simulink model "Traffic_Light_Final"  (R2016a)
settings: Solver=FixedStepDiscrete  StartTime=0.0  StopTime=inf  RelTol=1e-3
model workspace (MAT data in the model file):
  cs : Simulink.ConfigSet (value not decoded)
settings Model: Creator=LEGION  LastModifiedBy=LEGION
settings RTWCC: GenCodeOnly=on

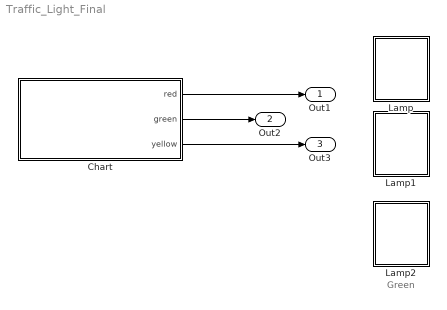
== system Traffic_Light_Final ==
  note: Green
  Chart : Stateflow chart  TreatAsAtomicUnit=on
  Lamp : Subsystem  DialogController=hmiCreateDDGDialog  IsWebBlock=on  mask(MWDashboardBlock){webBlockId=428b715c-2ac2-4c13-9f82-52b56b46ff5f, webBlockType=lamp, ShowInLibBrowser=on, ShowInitialText=on, HMISrcModelName=Traffic_Light_Final}
      mask prompts: webBlockType "WebBlock Type"; HMISrcModelName "Source Model"
      mask Help: helpview([docroot '/mapfiles/simulink.map'], 'hmi_lamp')
      mask Display:
      | if strcmp(get_param(bdroot(gcb),'BlockDiagramType'), 'library')
      |     image([(matlabroot) '/toolbox/simulink/hmi/icons/Lamp.png']);
      | end
  Lamp1 : Subsystem  DialogController=hmiCreateDDGDialog  IsWebBlock=on  mask(MWDashboardBlock){webBlockId=336aa306-1682-41f2-8291-8de665dc678f, webBlockType=lamp, ShowInLibBrowser=on, ShowInitialText=on, HMISrcModelName=Traffic_Light_Final}
      mask prompts: webBlockType "WebBlock Type"; HMISrcModelName "Source Model"
      mask Help: helpview([docroot '/mapfiles/simulink.map'], 'hmi_lamp')
      mask Display:
      | if strcmp(get_param(bdroot(gcb),'BlockDiagramType'), 'library')
      |     image([(matlabroot) '/toolbox/simulink/hmi/icons/Lamp.png']);
      | end
  Lamp2 : Subsystem  DialogController=hmiCreateDDGDialog  IsWebBlock=on  mask(MWDashboardBlock){webBlockId=cc7363f7-3161-4256-ad36-8951f7864fbc, webBlockType=lamp, ShowInLibBrowser=on, ShowInitialText=on, HMISrcModelName=Traffic_Light_Final}
      mask prompts: webBlockType "WebBlock Type"; HMISrcModelName "Source Model"
      mask Help: helpview([docroot '/mapfiles/simulink.map'], 'hmi_lamp')
      mask Display:
      | if strcmp(get_param(bdroot(gcb),'BlockDiagramType'), 'library')
      |     image([(matlabroot) '/toolbox/simulink/hmi/icons/Lamp.png']);
      | end
  Out1 : Outport
  Out2 : Outport  Port=2
  Out3 : Outport  Port=3
  wires:
  Chart/1(red) -> Out1/1
  Chart/2(green) -> Out2/1
  Chart/3(yellow) -> Out3/1

== system Traffic_Light_Final/Lamp ==

== system Traffic_Light_Final/Lamp1 ==

== system Traffic_Light_Final/Lamp2 ==

== stateflow chart Traffic_Light_Final/Chart ==
  state STOP
    entry:
    red=1;
    yellow=0;
    green=0;
  state PrepareToStop
    entry:
    red=0;
    yellow=1;
    green=0;
  state GO
    entry:
    red=0;
    yellow=0;
    green=1;
  (default) -> STOP
  STOP -> PrepareToStop : after(10,tick)
  PrepareToStop -> GO : after(3,tick)
  GO -> STOP : after(10,tick)
  data: red output; green output; yellow output
